simulink model "AEBS_decision_HWK7"  (R2023a)
settings: Solver=ode45  StartTime=0.0  StopTime=100  RelTol=1e-3
libraries: simulink x1, slpidlib x1
settings Model: Creator=Santo  LastModifiedBy=brianlesko
settings SolverCC: AlgebraicLoopSolver=TrustRegion
settings DataIOCC: ReturnWorkspaceOutputs=off
settings OptimizationCC: LifeSpan=inf
settings DebuggingCC: UnconnectedInputMsg=warning  UnconnectedOutputMsg=warning  UnconnectedLineMsg=warning  ArithmeticOperatorsInVariantConditions=warning
settings HardwareCC: ProdBitPerSizeT=32  ProdBitPerPtrDiffT=32  ProdWordSize=32  ProdHWDeviceType=Specified
settings ModelReferenceCC: EnableRefExpFcnMdlSchedulingChecks=on
settings SFSimCC: SimUseLocalCustomCode=off  CustomCodeUndefinedFunction=UseInterfaceOnly
settings RTWCC: RTWUseLocalCustomCode=off
settings CodeAppCC: StateflowObjectComments=on

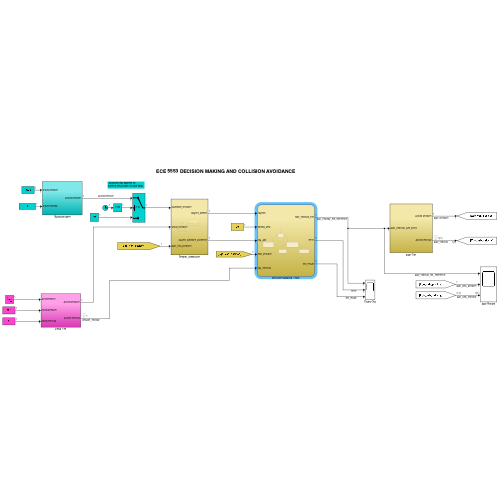
[thumbnail: Simulink's stored preview of the top-level diagram]
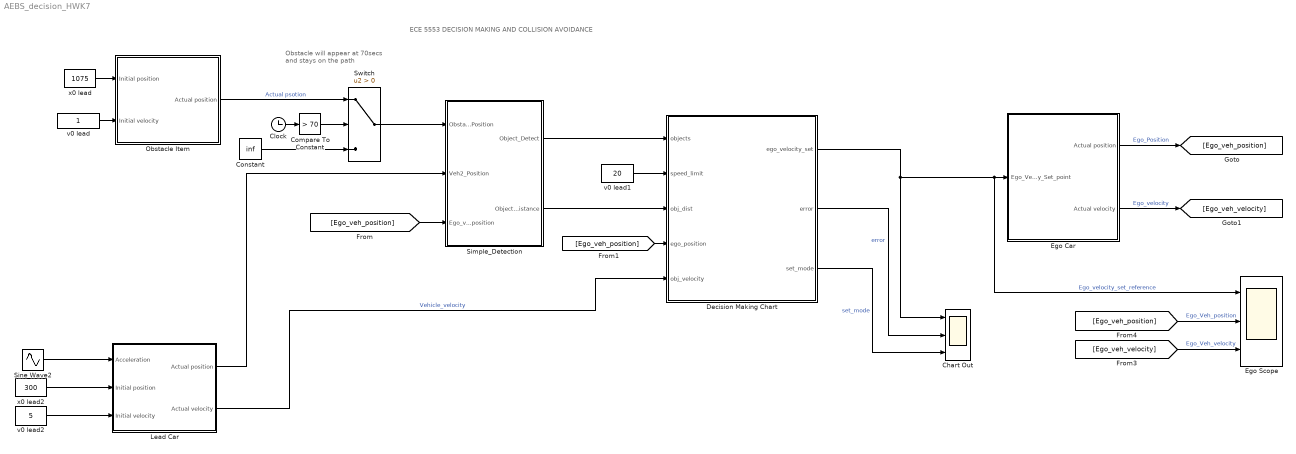
== system AEBS_decision_HWK7 ==
  note: ECE 5553 DECISION MAKING AND COLLISION AVOIDANCE
  note: Obstacle will appear at 70secs and stays on the path
  Chart Out : Scope  NumInputPorts=3
  Clock : Clock
  Compare To Constant : simulink/Logic and Bit Operations/Compare To Constant  relop=>  const=70  OutDataTypeStr=boolean
  Constant : Constant  Value=inf
  Decision Making Chart : Stateflow chart  TreatAsAtomicUnit=on
  Ego Car : Subsystem
  Ego Scope : Scope  NumInputPorts=3
  Lead Car : Subsystem
  Obstacle Item : Subsystem
  Simple_Detection : Subsystem
  Sine Wave2 : Sin  Amplitude=5  Frequency=0.5  SampleTime=0
  Switch : Switch  Criteria=u2 > Threshold  SaturateOnIntegerOverflow=off  InputSameDT=off
  v0 lead : Constant  SampleTime=0
  v0 lead1 : Constant  Value=20  SampleTime=0
  v0 lead2 : Constant  Value=5  SampleTime=0
  x0 lead : Constant  Value=1075  SampleTime=0
  x0 lead2 : Constant  Value=300  SampleTime=0
  wires:
  x0 lead/1 -> Obstacle Item/1(Initial position)
  v0 lead/1 -> Obstacle Item/2(Initial velocity)
  Lead Car/1(Actual position) -> Simple_Detection/2(Veh2_Position)
  x0 lead2/1 -> Lead Car/2(Initial position)
  v0 lead2/1 -> Lead Car/3(Initial velocity)
  Sine Wave2/1 -> Lead Car/1(Acceleration)
  Simple_Detection/1(Object_Detect) -> Decision Making Chart/1(objects)
  v0 lead1/1 -> Decision Making Chart/2(speed_limit)
  Decision Making Chart/1(ego_velocity_set) -> Chart Out/1, Ego Scope/1, Ego Car/1(Ego_Velocity_Set_point)  "Ego_velocity_set_reference"
  Ego Car/1(Actual position) -> [Ego_veh_position]  "Ego_Position"
  Ego Car/2(Actual velocity) -> [Ego_veh_velocity]  "Ego_velocity"
  Simple_Detection/2(Object_Relative_Distance) -> Decision Making Chart/3(obj_dist)
  Decision Making Chart/2(error) -> Chart Out/2  "error"
  [Ego_veh_position] -> Simple_Detection/3(Ego_veh_position)
  [Ego_veh_position] -> Decision Making Chart/4(ego_position)
  [Ego_veh_velocity] -> Ego Scope/3  "Ego_Veh_velocity"
  [Ego_veh_position] -> Ego Scope/2  "Ego_Veh_position"
  Decision Making Chart/3(set_mode) -> Chart Out/3  "set_mode"
  Lead Car/2(Actual velocity) -> Decision Making Chart/5(obj_velocity)  "Vehicle_velocity"
  Compare To Constant/1 -> Switch/2
  Switch/1 -> Simple_Detection/1(Obstacle_Position)
  Obstacle Item/1(Actual position) -> Switch/1  "Actual psotion"
  Constant/1 -> Switch/3
  Clock/1 -> Compare To Constant/1

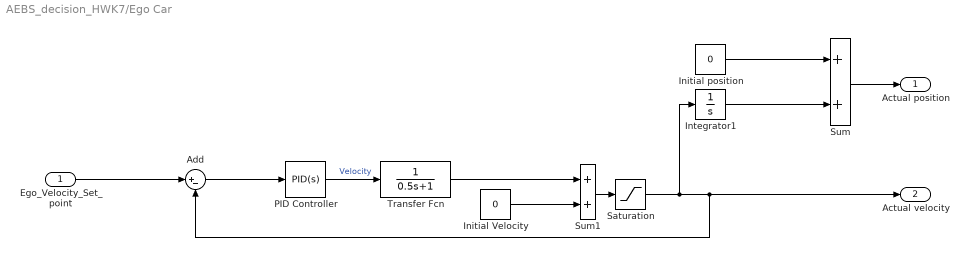
== system AEBS_decision_HWK7/Ego Car ==
  Ego_Velocity_Set_point : Inport
  Add : Sum  Inputs=|+-
  Initial Velocity : Constant  Value=0
  Initial position : Constant  Value=0
  Integrator1 : Integrator
  PID Controller : slpidlib/PID Controller  Controller=PID  Form=Parallel  TimeDomain=Continuous-time  UseExternalTs=off  SampleTime=-1  IntegratorMethod=Forward Euler  FilterMethod=Forward Euler  ControllerParametersSource=internal  P=0.543871188851985  I=1.5579001255467  UseKiTs=off  D=0  N=100  UseFilter=on  TunerSelectOption=Transfer Function Based (PID Tuner App)  InitialConditionSource=internal  InitialConditionForIntegrator=0  InitialConditionForFilter=0  DifferentiatorICPrevScaledInput=0  ExternalReset=none  TrackingMode=off  Kt=1  LimitOutput=off  SatLimitsSource=internal  UpperSaturationLimit=inf  LowerSaturationLimit=-inf  LinearizeAsGain=on  AntiWindupMode=none  Kb=1  LimitIntegrator=off  UpperIntegratorSaturationLimit=inf  LowerIntegratorSaturationLimit=-inf  POutMin=[]  POutMax=[]  IOutMin=[]  IOutMax=[]  DOutMin=[]  DOutMax=[]  NOutMin=[]  NOutMax=[]  SumOutMin=[]  SumOutMax=[]  SaturationOutMin=[]  SaturationOutMax=[]  PParamMin=[]  PParamMax=[]  IParamMin=[]  IParamMax=[]  DParamMin=[]  DParamMax=[]  NParamMin=[]  NParamMax=[]  KbParamMin=[]  KbParamMax=[]  KtParamMin=[]  KtParamMax=[]  KbOutMin=[]  KbOutMax=[]  KtOutMin=[]  KtOutMax=[]  IntegratorOutMin=[]  IntegratorOutMax=[]  FilterOutMin=[]  FilterOutMax=[]  SumI1OutMin=[]  SumI1OutMax=[]  SumI2OutMin=[]  SumI2OutMax=[]  SumI3OutMin=[]  SumI3OutMax=[]  SumI4OutMin=[]  SumI4OutMax=[]  SumDOutMin=[]  SumDOutMax=[]  DifferentiatorOutMin=[]  DifferentiatorOutMax=[]  FilterDiffOutCoefMin=[]  FilterDiffOutCoefMax=[]  ReciprocalOutMin=[]  ReciprocalOutMax=[]  SumDenOutMin=[]  SumDenOutMax=[]  SumNumOutMin=[]  SumNumOutMax=[]  DivideOutMin=[]  DivideOutMax=[]  UdiffTsProdOutMin=[]  UdiffTsProdOutMax=[]  NTsProdOutMin=[]  NTsProdOutMax=[]  UintegralTsProdOutMin=[]  UintegralTsProdOutMax=[]  UngainTsProdOutMin=[]  UngainTsProdOutMax=[]  ClampingZeroOutDataTypeStr=Inherit: Inherit via back propagation  ClampingZeroOutMin=[]  ClampingZeroOutMax=[]  FilterDenConstantOutDataTypeStr=Inherit: Inherit via back propagation  FilterDenConstantOutMin=[]  FilterDenConstantOutMax=[]  PCopyOutDataTypeStr=Inherit: Inherit via back propagation  PCopyOutMin=[]  PCopyOutMax=[]  NCopyOutDataTypeStr=Inherit: Inherit via back propagation  NCopyOutMin=[]  NCopyOutMax=[]  IntegratorContinuousStateAttributes=''  IntegratorStateMustResolveToSignalObject=off  IntegratorRTWStateStorageClass=Auto  FilterContinuousStateAttributes=''  FilterStateMustResolveToSignalObject=off  FilterRTWStateStorageClass=Auto  ParallelPVariant=InternalParameters  IdealPVariant=Disabled  IVariant=InternalParameters  DVariant=InternalParameters  IntegratorVariant=Continuous  SatVariant=Disabled  AWVariant=Passthrough  PCopyVariant=Disabled  TRVariant=Disabled  FdbkBlocksVariant=Forward  IdealPFdbkVariant=Disabled  SatFdbkVariant=Disabled  DerivativeFilterVariant=ContFilter  NVariant=InternalParameters  NCopyVariant=Disabled  FilterICVariant=InternalICsFilter  IntegratorICVariant=InternalICs  ExternalResetVariant=Disabled  TRSumVariant=Passthrough  SumFdbkVariant=Disabled  SumVariant=Sum_PID  TsampFilterVariant=InternalTs  TsampNgainVariant=Passthrough  TsampIntegralVariant=Disabled_SignalSpec  ExternalSaturationOutDataTypeStr=Inherit: Same as second input
  Saturation : Saturate  UpperLimit=inf  LowerLimit=0
  Sum : Sum
  Sum1 : Sum
  Transfer Fcn : TransferFcn  Denominator=[0.5 1]
  Actual position : Outport
  Actual velocity : Outport  Port=2
  wires:
  Transfer Fcn/1 -> Sum1/1
  Initial Velocity/1 -> Sum1/2
  Sum/1 -> Actual position/1
  Sum1/1 -> Saturation/1
  PID Controller/1 -> Transfer Fcn/1  "Velocity"
  Initial position/1 -> Sum/1
  Integrator1/1 -> Sum/2
  Add/1 -> PID Controller/1
  Ego_Velocity_Set_point/1 -> Add/1
  Saturation/1 -> Integrator1/1, Add/2, Actual velocity/1

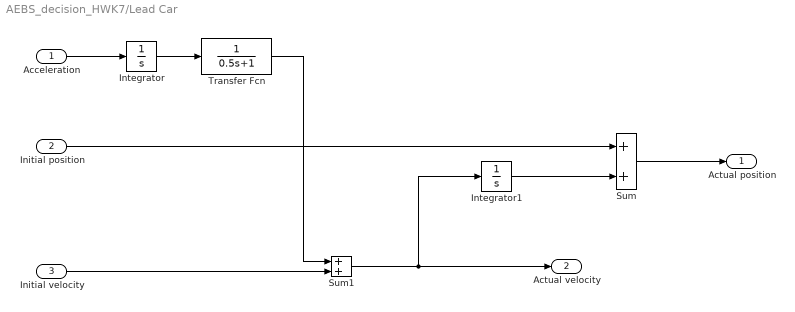
== system AEBS_decision_HWK7/Lead Car ==
  Acceleration : Inport
  Initial position : Inport  Port=2
  Initial velocity : Inport  Port=3
  Integrator : Integrator
  Integrator1 : Integrator
  Sum : Sum
  Sum1 : Sum
  Transfer Fcn : TransferFcn  Denominator=[0.5 1]
  Actual position : Outport
  Actual velocity : Outport  Port=2
  wires:
  Integrator1/1 -> Sum/2
  Initial position/1 -> Sum/1
  Acceleration/1 -> Integrator/1
  Sum1/1 -> Actual velocity/1, Integrator1/1
  Integrator/1 -> Transfer Fcn/1
  Sum/1 -> Actual position/1
  Initial velocity/1 -> Sum1/2
  Transfer Fcn/1 -> Sum1/1

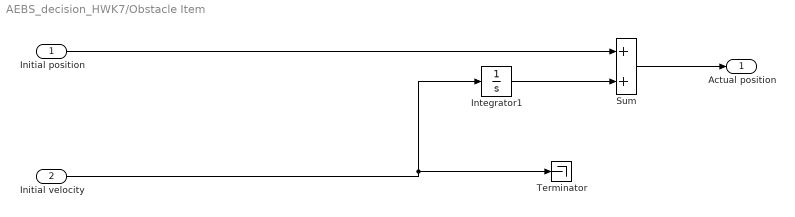
== system AEBS_decision_HWK7/Obstacle Item ==
  Initial position : Inport
  Initial velocity : Inport  Port=2
  Integrator1 : Integrator
  Sum : Sum
  Terminator : Terminator
  Actual position : Outport
  wires:
  Sum/1 -> Actual position/1
  Initial velocity/1 -> Terminator/1, Integrator1/1
  Initial position/1 -> Sum/1
  Integrator1/1 -> Sum/2

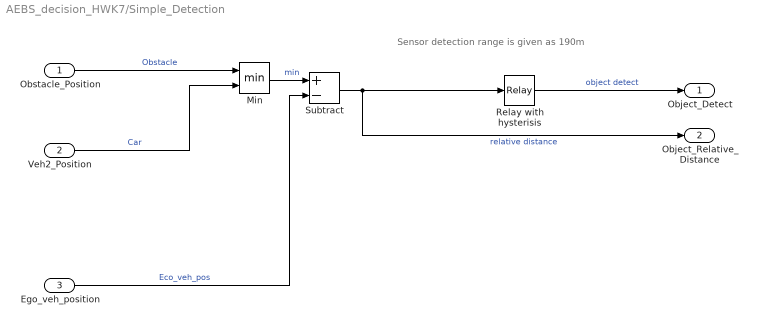
== system AEBS_decision_HWK7/Simple_Detection ==
  note: Sensor detection range is given as 190m
  Obstacle_Position : Inport
  Veh2_Position : Inport  Port=2
  Ego_veh_position : Inport  Port=3
  Min : MinMax  Inputs=2
  Relay with hysterisis : Relay  OnSwitchValue=210  OffSwitchValue=190  OnOutputValue=0  OffOutputValue=1
  Subtract : Sum  Inputs=+-
  Object_Detect : Outport
  Object_Relative_Distance : Outport  Port=2
  wires:
  Obstacle_Position/1 -> Min/1  "Obstacle"
  Veh2_Position/1 -> Min/2  "Car"
  Min/1 -> Subtract/1  "min"
  Ego_veh_position/1 -> Subtract/2  "Eco_veh_pos"
  Subtract/1 -> Relay with hysterisis/1, Object_Relative_Distance/1  "relative distance"
  Relay with hysterisis/1 -> Object_Detect/1  "object detect"

== stateflow chart AEBS_decision_HWK7/Decision Making Chart ==
  state Object_present
  state follow_speed_limit
    Ego_velocity = Speedlimit;
    set_mode = 0;
    error = 0;
  state set_error_to_distance_to_obstacle
    error = obj_dist;
    Ego_velocity = Speedlimit;
  state emergency_stop
    Ego_velocity = 0;
    set_mode = 2;
  state set_to_lead_car_vel
    Ego_velocity = obj_velocity;
    set_mode = 1;
  (default) -> Object_present
  Object_present -> follow_speed_limit [order 1] : [Object_Detect <1]
  Object_present -> set_error_to_distance_to_obstacle [order 2] : [Object_Detect == 1]
  set_error_to_distance_to_obstacle -> emergency_stop [order 1] : [error < 50]
  set_error_to_distance_to_obstacle -> set_to_lead_car_vel [order 2] : [error > 50]
  data: objects input; speed_limit input; ego_velocity_set output; obj_dist input; ego_position input; error output; set_mode output; obj_velocity input
